simulink model "keyonkeyoff"  (R2018b)
settings: Solver=VariableStepAuto  StartTime=0.0  StopTime=10.0  RelTol=1e-3
libraries: simulink x1, simulink_extras x1
settings Model: Creator=teus  LastModifiedBy=teus

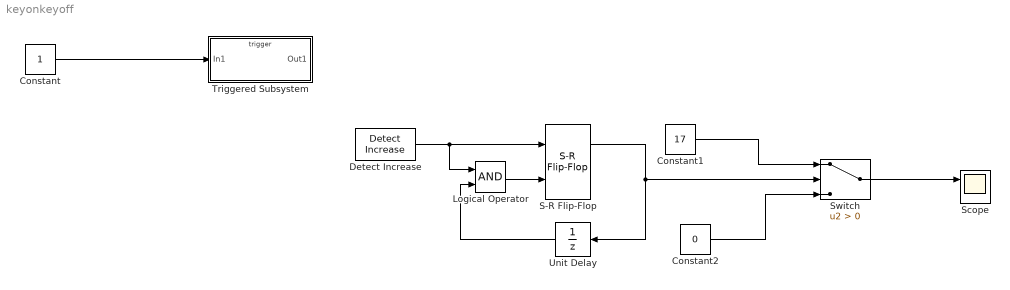
== system keyonkeyoff ==
  Constant : Constant  OutDataTypeStr=boolean
  Constant1 : Constant  Value=17
  Constant2 : Constant  Value=0
  Detect Increase : simulink/Logic and Bit Operations/Detect Increase  vinit=0.0  OutDataTypeStr=boolean
  Logical Operator : Logic  AllPortsSameDT=off  OutDataTypeStr=boolean
  S-R Flip-Flop : simulink_extras/Flip Flops/S-R Flip-Flop  initial_condition=0
  Scope : Scope  NumInputPorts=2
  Switch : Switch  Criteria=u2 > Threshold
  Triggered Subsystem : Subsystem  TreatAsAtomicUnit=on
  Unit Delay : UnitDelay  SampleTime=-1
  wires:
  Constant/1 -> Triggered Subsystem/1(In1)
  Logical Operator/1 -> S-R Flip-Flop/2
  S-R Flip-Flop/1 -> Switch/2, Unit Delay/1
  Unit Delay/1 -> Logical Operator/2
  Detect Increase/1 -> Logical Operator/1, S-R Flip-Flop/1
  Constant1/1 -> Switch/1
  Constant2/1 -> Switch/3
  Switch/1 -> Scope/1

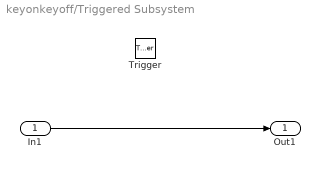
== system keyonkeyoff/Triggered Subsystem ==
  In1 : Inport
  Trigger : TriggerPort  TriggerType=either  VariantControl=Variant
  Out1 : Outport
  wires:
  In1/1 -> Out1/1
